simulink model "receiver_week12"  (R2022a)
settings: Solver=VariableStepAuto  StartTime=0.0  StopTime=inf  RelTol=1e-3
libraries: instrumentseriallib x2
settings Model: Creator=Reaper  LastModifiedBy=Reaper

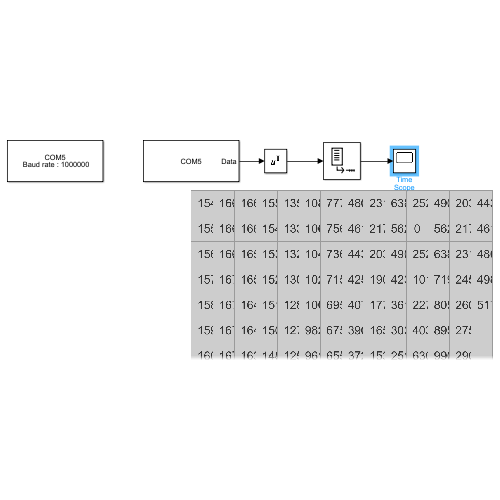
[thumbnail: Simulink's stored preview of the top-level diagram]
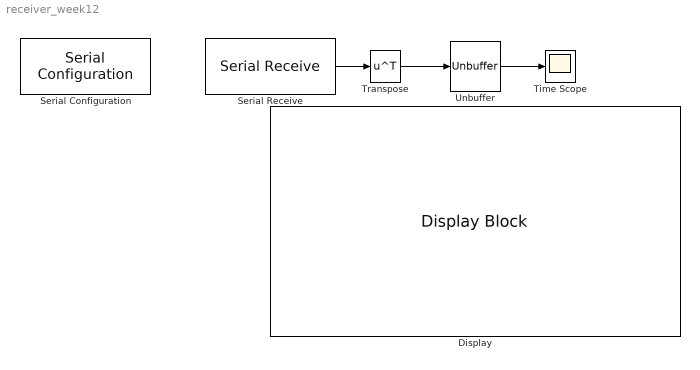
== system receiver_week12 ==
  Display : DisplayBlock  LabelPosition=Hide  Format=Integer  Transparency=1  Layout=Fill available space
  Serial Configuration : instrumentseriallib/Serial Configuration  Priority=-200000  PortSel=COM5  Port=COM5  ComPort=COM5  BaudRate=1000000  DataBits=8  Parity=none  StopBits=1  ByteOrder=little-endian  FlowControl=none  Timeout=10  SimulateUsing=Interpreted execution  BlockInModel=on  aMode=1
      settings: SourceProductBaseCode=OT,IC,MT
  Serial Receive : instrumentseriallib/Serial Receive  Priority=1  PortSel=COM5  Port=COM5  ComPort=COM5  DataType=uint32  SaveDataType=uint8  ToggleHeader=on  Header=[83 83]  ToggleTerminator=on  Terminator=Custom terminator  CustomTerminator=[69 69]  InputFormat=Column major  ToggleDataSize=on  DataSize=[1 1000]  EnableBlockingMode=on  ActionDataUnavailable=Output last received value  ActionWhenDataUnavailable=Output last received value  CustomValue=0  SampleTime=0.2  SimulateUsing=Interpreted execution  BlockInModel=on  aMode=1
      settings: SourceProductBaseCode=OT,IC,MT
  Time Scope : Scope
  Transpose : Math  Operator=transpose
  Unbuffer : Unbuffer
  wires:
  Serial Receive/1 -> Transpose/1
  Transpose/1 -> Unbuffer/1
  Unbuffer/1 -> Time Scope/1
